simulink model "assignment_1"  (R2017b)
settings: Solver=VariableStepAuto  StartTime=0.0  StopTime=10  FixedStep=0.001  RelTol=1e-6
values from neighbouring files (symbols this model uses):
  c1 = 17    [lab2_ass_variables.m]
  c2 = 1.2    [lab2_ass_variables.m]
  k1 = 0    [lab2_ass_variables.m]
  k2 = 390    [lab2_ass_variables.m]
  k3 = 0    [lab2_ass_variables.m]
  m1 = 2.77    [lab2_ass_variables.m]
  m2 = 2.59    [lab2_ass_variables.m]
settings Model: Creator=Tom Evetts  LastModifiedBy=Tom Evetts

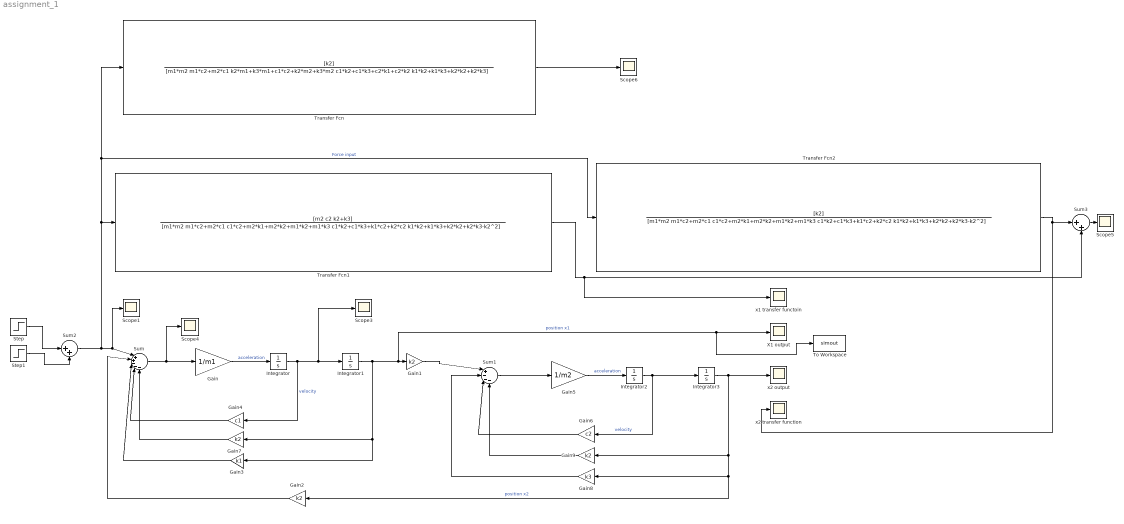
== system assignment_1 ==
  Gain : Gain  Gain=1/m1
  Gain{1..2,7,9} (4 alike) : Gain  Gain=k2
  Gain3 : Gain  Gain=k1
  Gain4 : Gain  Gain=c1
  Gain5 : Gain  Gain=1/m2
  Gain6 : Gain  Gain=c2
  Gain8 : Gain  Gain=k3
  Integrator{,1..3} (4 alike) : Integrator
  Scope{1,3..6} (5 alike) : Scope
  Step : Step  Time=0  After=20  SampleTime=0
  Step1 : Step  Time=0.025  After=-20  SampleTime=0
  Sum : Sum  Inputs=|++---
  Sum1 : Sum  Inputs=|+---
  Sum2 : Sum  Inputs=|++
  Sum3 : Sum  Inputs=|++
  To Workspace : ToWorkspace  VariableName=simout  SaveFormat=Timeseries  SampleTime=-1
  Transfer Fcn : TransferFcn  Numerator=[k2]  Denominator=[m1*m2 m1*c2+m2*c1 k2*m1+k3*m1+c1*c2+k2*m2+k3*m2 c1*k2+c1*k3+c2*k1+c2*k2 k1*k2+k1*k3+k2*k2+k2*k3]
  Transfer Fcn1 : TransferFcn  Numerator=[m2 c2 k2+k3]  Denominator=[m1*m2 m1*c2+m2*c1 c1*c2+m2*k1+m2*k2+m1*k2+m1*k3 c1*k2+c1*k3+k1*c2+k2*c2 k1*k2+k1*k3+k2*k2+k2*k3-k2^2]
  Transfer Fcn2 : TransferFcn  Numerator=[k2]  Denominator=[m1*m2 m1*c2+m2*c1 c1*c2+m2*k1+m2*k2+m1*k2+m1*k3 c1*k2+c1*k3+k1*c2+k2*c2 k1*k2+k1*k3+k2*k2+k2*k3-k2^2]
  X1 output : Scope
  x1 transfer functoin : Scope
  "x2 output " : Scope
  x2 transfer function : Scope
  wires:
  Step/1 -> Sum2/1
  Step1/1 -> Sum2/2
  Sum/1 -> Scope4/1, Gain/1
  Gain/1 -> Integrator/1  "acceleration"
  Sum2/1 -> Transfer Fcn2/1, Transfer Fcn/1, Transfer Fcn1/1, Sum/1, Scope1/1  "Force input"
  Integrator/1 -> Gain4/1, Scope3/1, Integrator1/1  "velocity"
  Gain1/1 -> Sum1/1
  Integrator1/1 -> Gain7/1, Gain3/1, To Workspace/1, X1 output/1, Gain1/1  "position x1"
  Gain3/1 -> Sum/3
  Gain4/1 -> Sum/4
  Sum1/1 -> Gain5/1
  Integrator2/1 -> Gain6/1, Integrator3/1  "velocity"
  Integrator3/1 -> Gain9/1, Gain8/1, Gain2/1, "x2 output "/1  "position x2"
  Gain5/1 -> Integrator2/1  "acceleration"
  Gain6/1 -> Sum1/3
  Gain8/1 -> Sum1/2
  Gain2/1 -> Sum/2
  Transfer Fcn/1 -> Scope6/1
  Transfer Fcn1/1 -> x1 transfer functoin/1, Sum3/2
  Sum3/1 -> Scope5/1
  Transfer Fcn2/1 -> Sum3/1, x2 transfer function/1
  Gain7/1 -> Sum/5
  Gain9/1 -> Sum1/4
